simulink model "Water_temp_changes"  (R2024b)
settings: Solver=VariableStepAuto  StartTime=0.0  StopTime=10.0  RelTol=1e-3
settings Model: Creator=kanith kumar  LastModifiedBy=kanith kumar

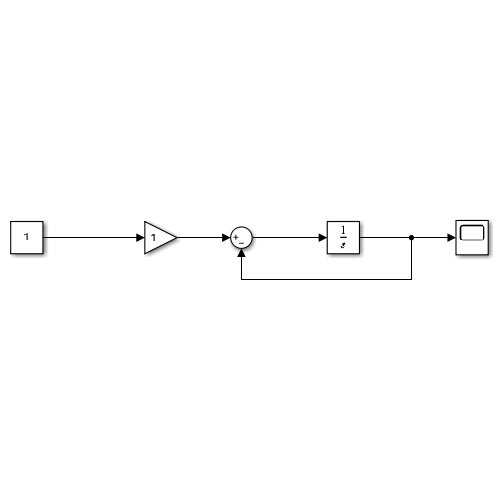
[thumbnail: Simulink's stored preview of the top-level diagram]
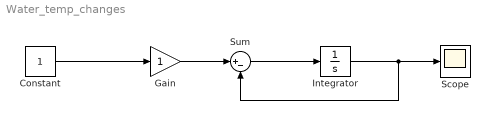
== system Water_temp_changes ==
  Constant : Constant
  Gain : Gain
  Integrator : Integrator
  Scope : Scope
  Sum : Sum  Inputs=|+-
  wires:
  Constant/1 -> Gain/1
  Integrator/1 -> Sum/2, Scope/1
  Gain/1 -> Sum/1
  Sum/1 -> Integrator/1
